simulink model "Question3"  (R2025a)
settings: Solver=VariableStepAuto  StartTime=0.0  StopTime=100  RelTol=1e-3
values from neighbouring files (symbols this model uses):
  d_Earth = -Pi_Luna * r_12    (= -4670658.19151)    [AER821_LAB_1.m]    (also in AER821_LAB_1_V2.m)
  d_Luna = Pi_Earth * r_12    (= 379729341.808)    [AER821_LAB_1.m]    (also in AER821_LAB_1_V2.m)
  Mu_Earth = G * M_Earth    (= 398716708000000)    [AER821_LAB_1.m]    (also in AER821_LAB_1_V2.m)
  Mu_Luna = G * M_Luna    (= 4904202160000)    [AER821_LAB_1.m]    (also in AER821_LAB_1_V2.m)
  Omega = sqrt(G * (M_Earth + M_Luna) / r_12^3)    [AER821_LAB_1.m]    (also in AER821_LAB_1_V2.m)
  r0x = xL1    [AER821_LAB_1.m]    (also in AER821_LAB_1_V2.m)
  r0y = 0    [AER821_LAB_1.m]    (also in AER821_LAB_1_V2.m)
  r0z = 0    [AER821_LAB_1.m]    (also in AER821_LAB_1_V2.m)
  r_earth = sqrt( (x-d_Earth)^2 + y^2 + z^2)    [AER821_LAB_1.m]    (also in AER821_LAB_1_V2.m = r0x - d_Earth)
  r_moon = sqrt( (x-d_Luna)^2 + y^2 + z^2)    [AER821_LAB_1.m]    (also in AER821_LAB_1_V2.m = d_Luna-r0x)
  v0x = 0    [AER821_LAB_1.m]    (also in AER821_LAB_1_V2.m)
  v0y = Omega * xL1    [AER821_LAB_1.m]    (also in AER821_LAB_1_V2.m)
  v0z = 0    [AER821_LAB_1.m]    (also in AER821_LAB_1_V2.m)
settings Model: Creator=User  LastModifiedBy=bosco
settings DebuggingCC: UnderSpecifiedDimensionMsg=error
settings RTWCC: GPUComputeCapability=3.5

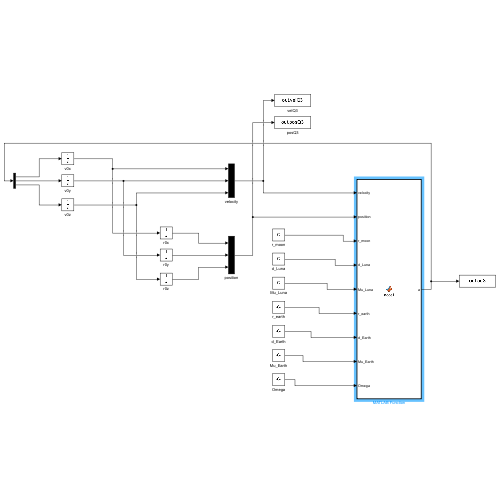
[thumbnail: Simulink's stored preview of the top-level diagram]
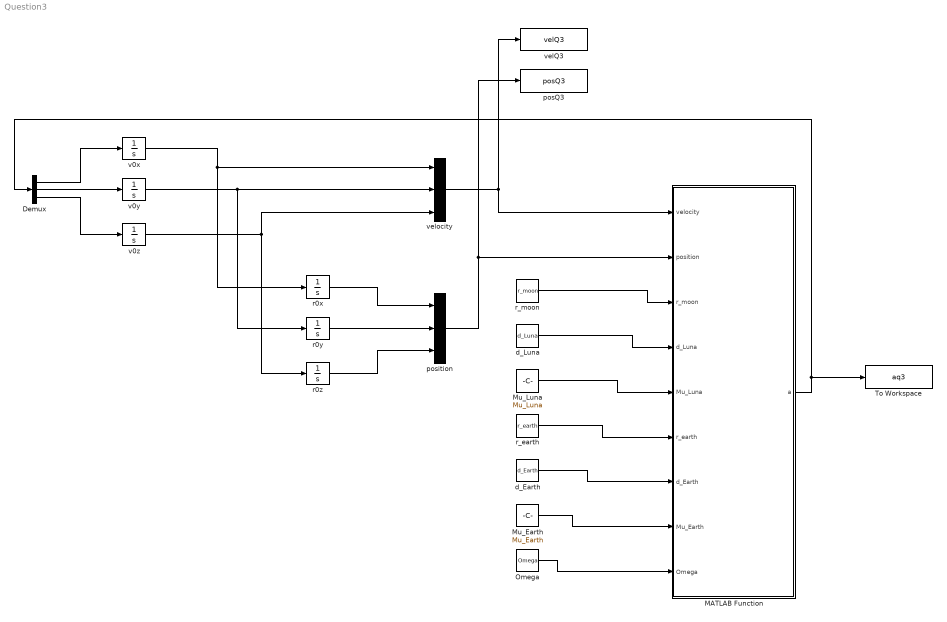
== system Question3 ==
  Demux : Demux  Outputs=3
  MATLAB Function : MATLAB Function  TreatAsAtomicUnit=on
  Mu_Earth : Constant  Value=Mu_Earth
  Mu_Luna : Constant  Value=Mu_Luna
  Omega : Constant  Value=Omega
  To Workspace : ToWorkspace  VariableName=aq3  SaveFormat=Timeseries  SampleTime=-1
  d_Earth : Constant  Value=d_Earth
  d_Luna : Constant  Value=d_Luna
  posQ3 : ToWorkspace  VariableName=posQ3  SaveFormat=Timeseries  SampleTime=-1
  position : Mux  Inputs=3
  r0x : Integrator  InitialCondition=r0x
  r0y : Integrator  InitialCondition=r0y
  r0z : Integrator  InitialCondition=r0z
  r_earth : Constant  Value=r_earth
  r_moon : Constant  Value=r_moon
  v0x : Integrator  InitialCondition=v0x
  v0y : Integrator  InitialCondition=v0y
  v0z : Integrator  InitialCondition=v0z
  velQ3 : ToWorkspace  VariableName=velQ3  SaveFormat=Timeseries  SampleTime=-1
  velocity : Mux  Inputs=3
  wires:
  Omega/1 -> MATLAB Function/9(Omega)
  Mu_Earth/1 -> MATLAB Function/8(Mu_Earth)
  d_Earth/1 -> MATLAB Function/7(d_Earth)
  r_earth/1 -> MATLAB Function/6(r_earth)
  Mu_Luna/1 -> MATLAB Function/5(Mu_Luna)
  d_Luna/1 -> MATLAB Function/4(d_Luna)
  r_moon/1 -> MATLAB Function/3(r_moon)
  MATLAB Function/1(a) -> Demux/1, To Workspace/1
  r0y/1 -> position/2
  r0x/1 -> position/1
  r0z/1 -> position/3
  v0y/1 -> r0y/1, velocity/2
  v0x/1 -> r0x/1, velocity/1
  v0z/1 -> velocity/3, r0z/1
  velocity/1 -> velQ3/1, MATLAB Function/1(velocity)
  position/1 -> posQ3/1, MATLAB Function/2(position)
  Demux/2 -> v0y/1
  Demux/1 -> v0x/1
  Demux/3 -> v0z/1

== matlab function Question3/MATLAB Function ==
  data: velocity input; position input; r_moon input; a output size=[3 1]; d_Luna input; Mu_Luna input; r_earth input; d_Earth input; Mu_Earth input; Omega input
function a = accel(velocity, position, r_moon, d_Luna, Mu_Luna, r_earth, d_Earth, Mu_Earth, Omega)

    %% Define variables
    
    % position
    x = position(1);
    y = position(2);
    z = position(3);
    
    % velocity
    x_v = velocity(1);
    y_v = velocity(2);


     
    %% Function
    
    ax = 2*Omega*y_v + (Omega^2)*x - (Mu_Earth / r_earth^3)*(x-d_Earth) - (Mu_Luna / r_moon^3)*(x-d_Luna);
    
    ay = -(Mu_Earth / r_earth^3)*y - (Mu_Luna / r_moon^3)*y + (Omega^2)*y - 2*Omega*x_v;
    
    az = -(Mu_Earth / r_earth^3)*z - (Mu_Luna / r_moon^3)*z;
    
    a = [ax; ay; az];
